simulink model "LQG_tw_v4"  (R2019a)
settings: Solver=FixedStepAuto  StartTime=0.0  StopTime=15  FixedStep=0.01  RelTol=1e-3
settings Model: Creator=chute  LastModifiedBy=chute
settings DataIOCC: ReturnWorkspaceOutputs=off

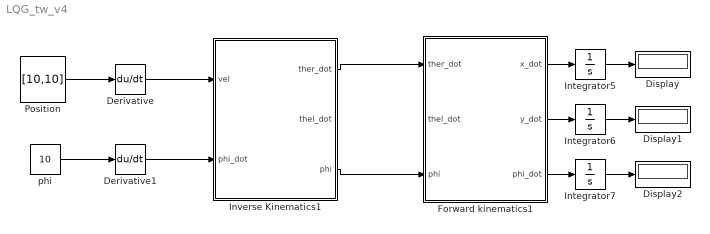
== system LQG_tw_v4 ==
  Derivative : Derivative
  Derivative1 : Derivative
  Display : Display
      settings: Decimation=3
  Display1 : Display
      settings: Decimation=3
  Display2 : Display
      settings: Decimation=3
  Forward kinematics1 : MATLAB Function  TreatAsAtomicUnit=on
  Integrator5 : Integrator
  Integrator6 : Integrator
  Integrator7 : Integrator  InitialCondition=[0;0]
  Inverse Kinematics1 : MATLAB Function  TreatAsAtomicUnit=on
  Position : Constant  Value=[10,10]
  phi : Constant  Value=10
  wires:
  Forward kinematics1/1(x_dot) -> Integrator5/1
  Integrator5/1 -> Display/1
  Integrator6/1 -> Display1/1
  Integrator7/1 -> Display2/1
  Forward kinematics1/2(y_dot) -> Integrator6/1
  Forward kinematics1/3(phi_dot) -> Integrator7/1
  Position/1 -> Derivative/1
  Derivative/1 -> Inverse Kinematics1/1(vel)
  Derivative1/1 -> Inverse Kinematics1/2(phi_dot)
  phi/1 -> Derivative1/1
  Inverse Kinematics1/1(ther_dot) -> Forward kinematics1/1(ther_dot)
  Inverse Kinematics1/3(phi) -> Forward kinematics1/3(phi)

== matlab function LQG_tw_v4/Forward kinematics1 ==
  data: ther_dot input; thel_dot input; x_dot output; y_dot output; phi_dot output; phi input
function [x_dot, y_dot,phi_dot] = FK(ther_dot,thel_dot,phi)
R =0.0335; % Wheel radius
W =0.17; % Body width

% thel_dot= (the_dot-(phi_dot*W)/R);
% ther_dot= the_dot+phi_dot*W/(2*R);

for i=1:1
    J=[(R/2)*cos(phi(i)),(R/2)*cos(phi(i));
       (R/2)*sin(phi(i)),(R/2)*sin(phi(i));
                     R/W,           -R/W];
end
out =J*[ther_dot;thel_dot];
x_dot=out(1,1);
y_dot =out(2,1);
phi_dot=out(3,1);
end

== matlab function LQG_tw_v4/Inverse Kinematics1 ==
  data: vel input; ther_dot output; thel_dot output; phi_dot input; phi output
function [ther_dot,thel_dot,phi]  = fcn(vel,phi_dot)

x_dot=vel(1,1);
y_dot=vel(2,1);
R =0.0335; % Wheel radius
W =0.17; % Body width
a=y_dot;
b=-x_dot;
d=0;
anp = atan2(b, a);
x1= anp + atan2(sqrt(a*a + b*b - d*d), d);
x2= anp + atan2(-sqrt(a*a + b*b - d*d), d);
phi  =[x1;x2];
    for i=1:2
        j=(1/R)*[cos(phi(i)),sin(phi(i)),W/(2);
                 cos(phi(i)),sin(phi(i)),-W/(2)];
        out1=j*[x_dot;y_dot;phi_dot(i)];
    end
ther_dot=out1(1,1);
thel_dot=out1(2,1);

% the_dot =(1/2)*(ther_dot+thel_dot);
